simulink model "Kalman"  (R2020b)
settings: Solver=VariableStepAuto  StartTime=0.0  StopTime=10.0  RelTol=1e-3
settings Model: Creator=danie  LastModifiedBy=danie

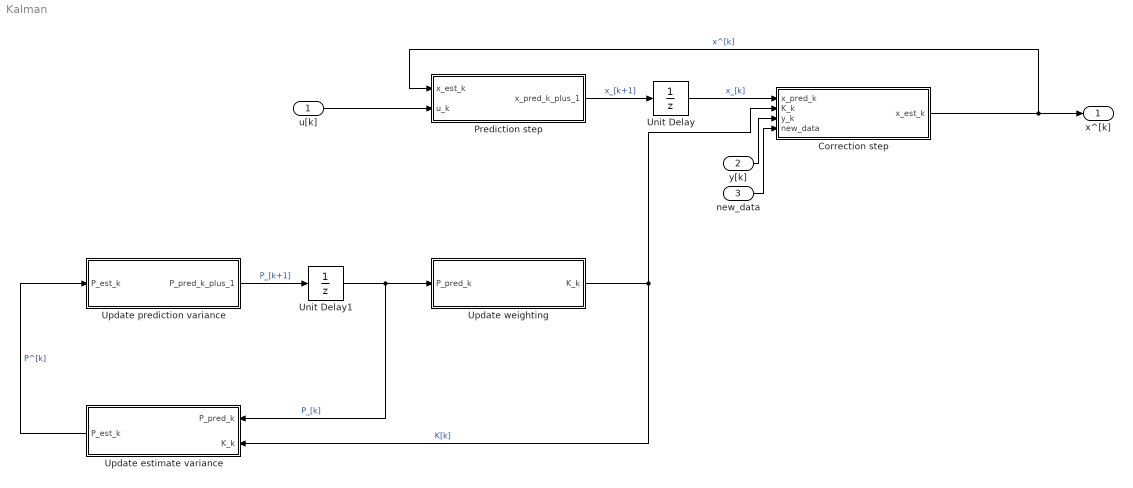
== system Kalman ==
  u[k] : Inport
  y[k] : Inport  Port=2
  new_data : Inport  Port=3
  Correction step : MATLAB Function  TreatAsAtomicUnit=on
  Prediction step : MATLAB Function  TreatAsAtomicUnit=on
  Unit Delay : UnitDelay  SampleTime=-1  HasFrameUpgradeWarning=on
  Unit Delay1 : UnitDelay  SampleTime=-1  HasFrameUpgradeWarning=on
  Update estimate variance : MATLAB Function  TreatAsAtomicUnit=on
  Update prediction variance : MATLAB Function  TreatAsAtomicUnit=on
  Update weighting : MATLAB Function  TreatAsAtomicUnit=on
  x^[k] : Outport
  wires:
  Correction step/1(x_est_k) -> Prediction step/1(x_est_k), x^[k]/1  "x^[k]"
  u[k]/1 -> Prediction step/2(u_k)
  Prediction step/1(x_pred_k_plus_1) -> Unit Delay/1  "x_[k+1]"
  Unit Delay/1 -> Correction step/1(x_pred_k)  "x_[k]"
  y[k]/1 -> Correction step/3(y_k)
  new_data/1 -> Correction step/4(new_data)
  Update prediction variance/1(P_pred_k_plus_1) -> Unit Delay1/1  "P_[k+1]"
  Unit Delay1/1 -> Update estimate variance/1(P_pred_k), Update weighting/1(P_pred_k)  "P_[k]"
  Update weighting/1(K_k) -> Correction step/2(K_k), Update estimate variance/2(K_k)  "K[k]"
  Update estimate variance/1(P_est_k) -> Update prediction variance/1(P_est_k)  "P^[k]"

== matlab function Kalman/Correction step ==
  data: x_pred_k input; x_est_k output; K_k input; y_k input; new_data input
function x_est_k = fcn(x_pred_k, K_k, y_k, new_data)
    if ~new_data
        x_est_k = x_pred_k;
    else
        x_est_k = x_pred_k + K_k*(y_k - C_d*x_pred_k);
    end

== matlab function Kalman/Prediction step ==
  data: x_est_k input; x_pred_k_plus_1 output; u_k input
function x_pred_k_plus_1 = fcn(x_est_k, u_k)
x_pred_k_plus_1 = A_d*x_est_k+B_d*u_k;

== matlab function Kalman/Update prediction variance ==
  data: P_est_k input; P_pred_k_plus_1 output
function P_pred_k_plus_1 = fcn(P_est_k)
P_pred_k_plus_1 = A_d*P_est_k*A_d' + Q_d;

== matlab function Kalman/Update weighting ==
  data: P_pred_k input; K_k output
function K_k = fcn(P_pred_k)
K_k = P_pred_k*C_d'*(C_d*P_pred_k*C_d' + R_d)^(-1);

== matlab function Kalman/Update estimate variance ==
  data: P_pred_k input; P_est_k output; K_k input
function P_est_k = fcn(P_pred_k, K_k)
temp = (eye(dim(K_k)) - K_k*C_d);
P_est_k = temp*P_pred_k*temp' + K_k*R_d*K_k';
